simulink model "m010_ConstAndDly"  (R2022a)
settings: Solver=VariableStepAuto  StartTime=0.0  StopTime=10.0  RelTol=1e-3
settings Model: Creator=Admin  LastModifiedBy=Admin

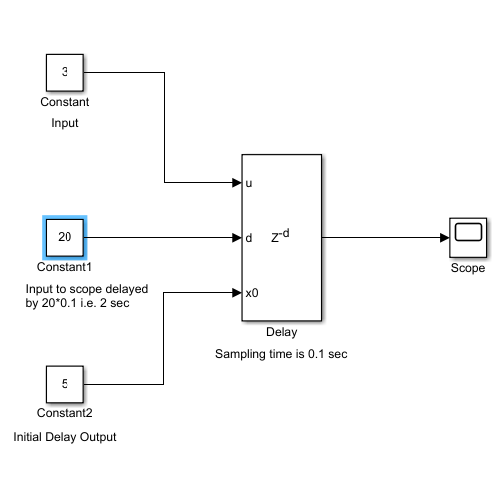
[thumbnail: Simulink's stored preview of the top-level diagram]
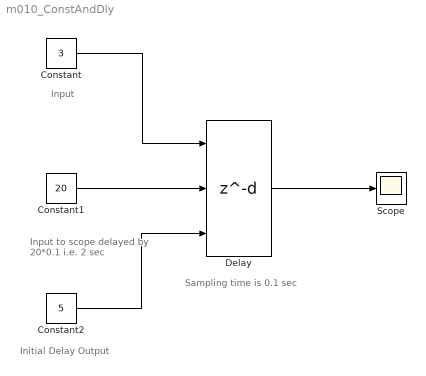
== system m010_ConstAndDly ==
  note: Input to scope delayed
      | by 20*0.1 i.e. 2 sec
  note: Input
  note: Initial Delay Output
  note: Sampling time is 0.1 sec
  Constant : Constant  Value=3
  Constant1 : Constant  Value=20
  Constant2 : Constant  Value=5
  Delay : Delay  DelayLengthSource=Input port  DelayLength=30  InitialConditionSource=Input port  InitialCondition=0  SampleTime=0.1
      settings: InputPortMap=u0,p1,p4
  Scope : Scope
  wires:
  Delay/1 -> Scope/1
  Constant/1 -> Delay/1
  Constant2/1 -> Delay/3
  Constant1/1 -> Delay/2
